simulink model "Central_Door_Locking_System"  (R2025a)
settings: Solver=VariableStepAuto  StartTime=0.0  StopTime=35  RelTol=1e-3
libraries: SignalEditorBlockLib x1
settings Model: Creator=Rudransh  LastModifiedBy=Rudransh

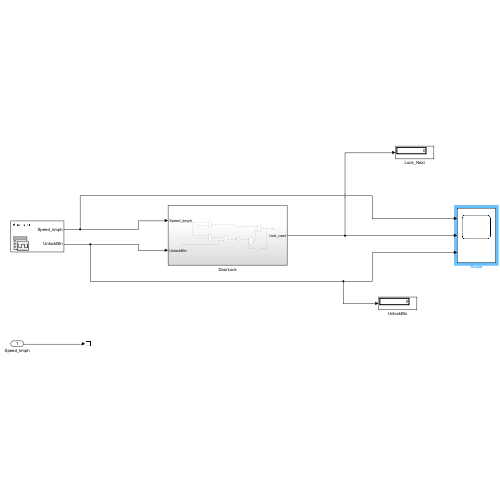
[thumbnail: Simulink's stored preview of the top-level diagram]
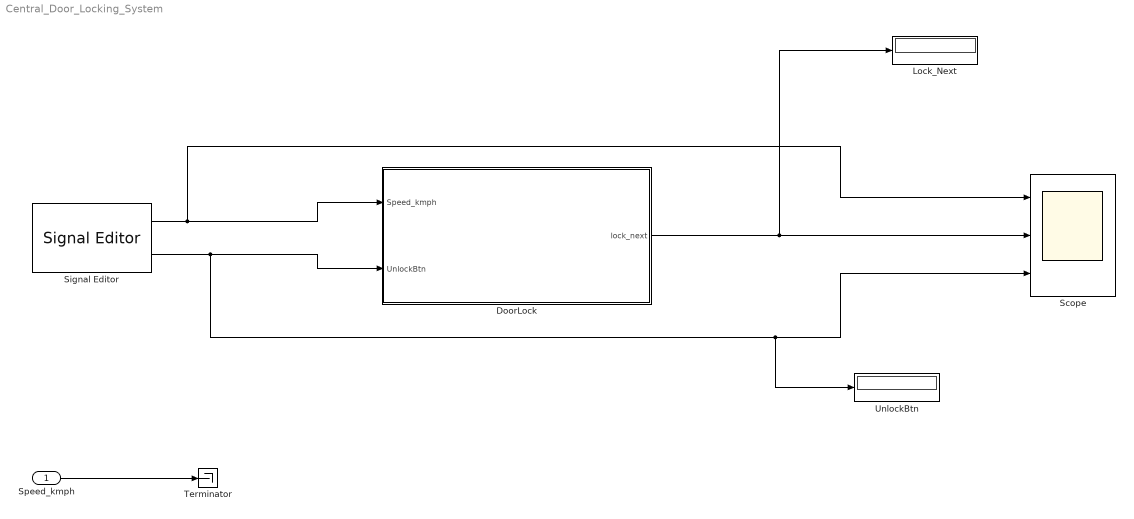
== system Central_Door_Locking_System ==
  Speed_kmph : Inport
  DoorLock : Subsystem
  Lock_Next : Display
  Scope : Scope  NumInputPorts=3
      settings: ActiveDisplayString=3  Title=UnlockBtn  ActiveDisplayYMinimum=0  ActiveDisplayYMaximum=1
  Signal Editor : SignalEditorBlockLib/Signal Editor  FileName=C:\Projects_ESD\AUTOSAR_CARSYSTEM\Central_Locking_System\Scenario\Scenario3.mat  ActiveScenario=Scenario  ActiveSignal=Speed_kmph  IsBus=off  OutputBusObjectStr=Bus: BusObject  SampleTime=0  ZeroCross=off  OutputAfterFinalValue=Setting to zero  Unit=inherit  PreserveSignalName=on  ApplySigPropsToAllScenarios=on  ApplySigPropsToAllSignals=off  SignalPropertySource=Dialog parameters
  Terminator : Terminator
  UnlockBtn : Display
  wires:
  Signal Editor/1 -> Scope/1, DoorLock/1(Speed_kmph)
  Signal Editor/2 -> UnlockBtn/1, Scope/3, DoorLock/2(UnlockBtn)
  Speed_kmph/1 -> Terminator/1
  DoorLock/1(lock_next) -> Lock_Next/1, Scope/2

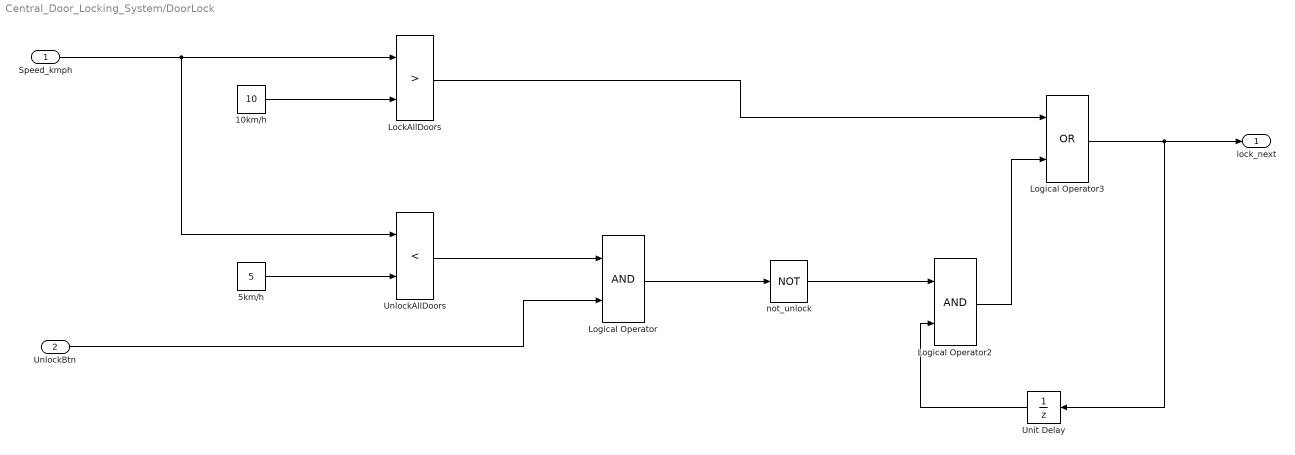
== system Central_Door_Locking_System/DoorLock ==
  Speed_kmph : Inport
  UnlockBtn : Inport  Port=2
  10km/h : Constant  Value=10
  5km/h : Constant  Value=5
  LockAllDoors : RelationalOperator  Operator=>  OutDataTypeStr=boolean  RndMeth=Simplest  InputSameDT=off
  Logical Operator : Logic  AllPortsSameDT=off  OutDataTypeStr=boolean
  Logical Operator2 : Logic  AllPortsSameDT=off  OutDataTypeStr=boolean
  Logical Operator3 : Logic  Operator=OR  AllPortsSameDT=off  OutDataTypeStr=boolean
  Unit Delay : UnitDelay  SampleTime=-1  HasFrameUpgradeWarning=on
  UnlockAllDoors : RelationalOperator  Operator=<  OutDataTypeStr=boolean  RndMeth=Simplest  InputSameDT=off
  not_unlock : Logic  Operator=NOT  AllPortsSameDT=off  OutDataTypeStr=boolean
  lock_next : Outport
  wires:
  Logical Operator2/1 -> Logical Operator3/2
  10km/h/1 -> LockAllDoors/2
  5km/h/1 -> UnlockAllDoors/2
  LockAllDoors/1 -> Logical Operator3/1
  Speed_kmph/1 -> UnlockAllDoors/1, LockAllDoors/1
  Logical Operator3/1 -> lock_next/1, Unit Delay/1
  Unit Delay/1 -> Logical Operator2/2
  UnlockAllDoors/1 -> Logical Operator/1
  UnlockBtn/1 -> Logical Operator/2
  Logical Operator/1 -> not_unlock/1
  not_unlock/1 -> Logical Operator2/1
